simulink model "Wiper_System_sim_model"  (R2023a)
settings: Solver=VariableStepAuto  StartTime=0.0  StopTime=10.0  RelTol=1e-3
settings Model: Creator=vaibh  LastModifiedBy=vaibh

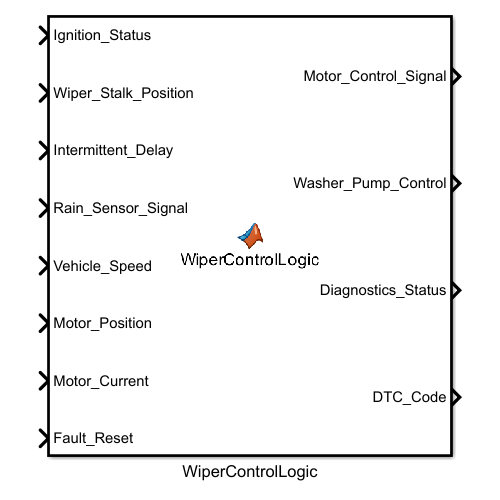
[thumbnail: Simulink's stored preview of the top-level diagram]
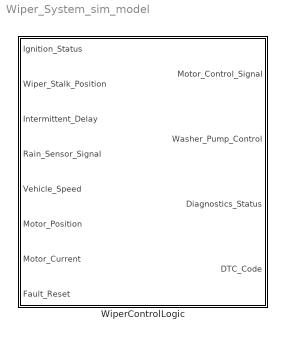
== system Wiper_System_sim_model ==
  WiperControlLogic : MATLAB Function  TreatAsAtomicUnit=on

== matlab function Wiper_System_sim_model/WiperControlLogic ==
  data: Ignition_Status input; Motor_Control_Signal output; Wiper_Stalk_Position input; Intermittent_Delay input; Rain_Sensor_Signal input; Vehicle_Speed input; Motor_Position input; Motor_Current input; Fault_Reset input; Washer_Pump_Control output; Diagnostics_Status output; DTC_Code output
function [Motor_Control_Signal, Washer_Pump_Control, Diagnostics_Status, DTC_Code] = ...
    WiperControlLogic(Ignition_Status, Wiper_Stalk_Position, Intermittent_Delay, ...
    Rain_Sensor_Signal, Vehicle_Speed, Motor_Position, Motor_Current, Fault_Reset)

    % Constants
    PARK_POSITION = 0;         % Motor park position
    MAX_CURRENT = 10.0;        % Max allowable current (in Amps)
    THRESHOLD_RAIN_LOW = 200;  % Rain intensity low threshold
    THRESHOLD_RAIN_HIGH = 800; % Rain intensity high threshold

    % Outputs - Initialization
    Motor_Control_Signal = 0;  % 0 = Stop, 1 = Low Speed, 2 = High Speed
    Washer_Pump_Control = false;
    Diagnostics_Status = 0;    % 0 = OK, 1 = Warning, 2 = Fault
    DTC_Code = 0;              % 0 = No Fault, 101 = Motor Stall, 102 = Overcurrent

    persistent motor_fault;    % Store fault state across function calls
    if isempty(motor_fault)
        motor_fault = false;
    end

    % Fault Reset Logic
    if Fault_Reset
        motor_fault = false;
        Diagnostics_Status = 0;
        DTC_Code = 0;
    end

    % If ignition is off, ensure motor is parked and return
    if Ignition_Status == 0
        if Motor_Position ~= PARK_POSITION
            Motor_Control_Signal = 1; % Run motor to park position
        else
            Motor_Control_Signal = 0; % Stop motor
        end
        return;
    end

    % Motor Current Fault Detection
    if Motor_Current > MAX_CURRENT
        motor_fault = true;
        Diagnostics_Status = 2; % Fault state
        DTC_Code = 102;         % Overcurrent Fault
        Motor_Control_Signal = 0; % Stop motor
        return;
    end

    % Wiper Stalk Position Handling
    switch Wiper_Stalk_Position
        case 0 % OFF
            if Motor_Position ~= PARK_POSITION
                Motor_Control_Signal = 1; % Move to park
            else
                Motor_Control_Signal = 0; % Stop motor
            end

        case 1 % LOW
            Motor_Control_Signal = 1; % Run motor at low speed

        case 2 % HIGH
            Motor_Control_Signal = 2; % Run motor at high speed

        case 3 % INTERMITTENT
            Motor_Control_Signal = 1; % Run motor for one cycle
            pause(Intermittent_Delay / 1000); % Delay in seconds
            Motor_Control_Signal = 0; % Stop motor

        case 4 % WASHER
            Washer_Pump_Control = true; % Activate washer pump
            Motor_Control_Signal = 1;  % Run motor at low speed
            pause(1);                  % Washer operation duration (1 sec)
            Washer_Pump_Control = false;
            Motor_Control_Signal = 0;

        otherwise
            Diagnostics_Status = 1;    % Warning state (Invalid stalk position)
            DTC_Code = 201;            % Invalid stalk position fault
    end

    % Rain Sensor Mode Handling
    if Wiper_Stalk_Position == 3 && Rain_Sensor_Signal > 0
        if Rain_Sensor_Signal > THRESHOLD_RAIN_HIGH
            Motor_Control_Signal = 2; % High speed
        elseif Rain_Sensor_Signal > THRESHOLD_RAIN_LOW
            Motor_Control_Signal = 1; % Low speed
        else
            Motor_Control_Signal = 0; % Stop motor
        end
    end

    % Motor Stall Detection
    if Motor_Control_Signal > 0 && Motor_Position == PARK_POSITION
        motor_fault = true;
        Diagnostics_Status = 2; % Fault state
        DTC_Code = 101;         % Motor stall fault
        Motor_Control_Signal = 0; % Stop motor
    end
end
